simulink model "sk_R3GDL"  (Simulink 9.0)
settings: Solver=ode45  StartTime=0.0  StopTime=Tsim  MaxStep=1e-3  RelTol=1e-3  EnableMultiTasking=on
values from neighbouring files (symbols this model uses):
  A_a = [0.1 0.1 0.1]    [Estimacion_de_Parametros.m]
  A_b = [0.5 0.5 0.5]    [Estimacion_de_Parametros.m]
  Im_cc = [0 1 0.5]    [Estimacion_de_Parametros.m]
  R1 = 50    [Estimacion_de_Parametros.m]
  R2 = 30    [Estimacion_de_Parametros.m]
  R3 = 15    [Estimacion_de_Parametros.m]
  tau = 7    [Estimacion_de_Parametros.m]
  Ts = 0.001    [Estimacion_de_Parametros.m]
  W_a = [15 15 15]    [Estimacion_de_Parametros.m]
  W_b = [3 6 6]    [Estimacion_de_Parametros.m]
settings Model: Creator=mortega  LastModifiedBy=Alvaro  ExtModeTrigMode=oneshot  ExtModeArmWhenConnect=off
settings DataIOCC: SignalLoggingSaveFormat=ModelDataLogs
settings OptimizationCC: BlockReduction=off  BooleanDataType=off  ExpressionDepthLimit=2147483647  InitFltsAndDblsToZero=on
settings DebuggingCC: SaveWithParameterizedLinksMsg=none  SignalResolutionControl=TryResolveAllWithWarning  MultiTaskDSMMsg=warning  MultiTaskCondExecSysMsg=none  FcnCallInpInsideContextMsg=warning  StateNameClashWarn=warning  StrictBusMsg=None
settings HardwareCC: TargetUnknown=on
settings GRTTargetCC: TargetFcnLib=ansi_tfl_tmw.mat  CombineOutputUpdateFcns=off  GRTInterface=on

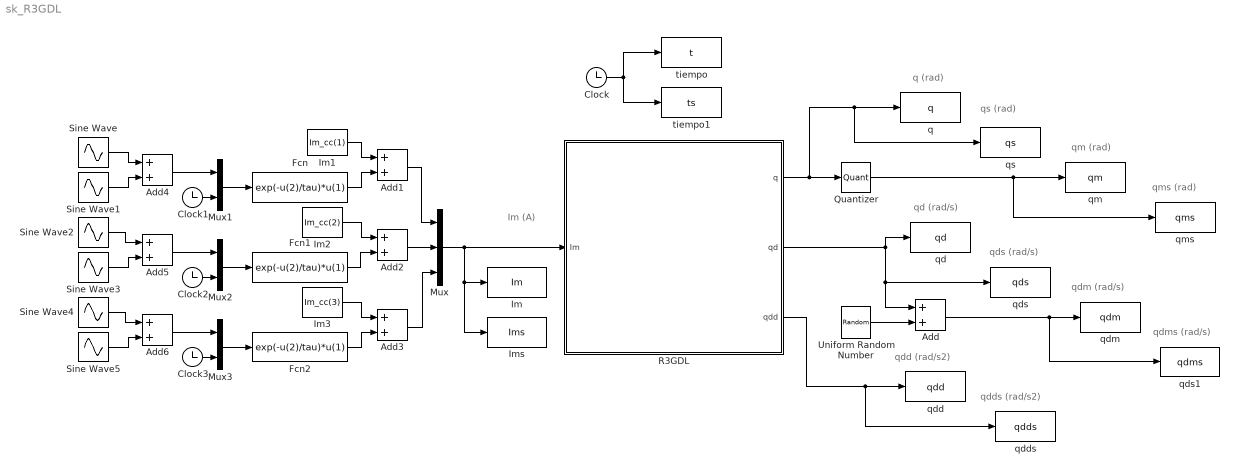
== system sk_R3GDL ==
  note: Im (A)
  note: q (rad)
  note: qd (rad/s)
  note: qdd (rad/s2)
  note: qs (rad)
  note: qds (rad/s)
  note: qdds (rad/s2)
  note: qm (rad)
  note: qms (rad)
  note: qdm (rad/s)
  note: qdms (rad/s)
  Add{,1..6} (7 alike) : Sum
  Clock{,1..3} (4 alike) : Clock
  Fcn : Fcn  Expr=exp(-u(2)/tau)*u(1)
  Fcn1 : Fcn  Expr=exp(-u(2)/tau)*u(1)
  Fcn2 : Fcn  Expr=exp(-u(2)/tau)*u(1)
  Im : ToWorkspace  VariableName=Im  SampleTime=-1
  Im1 : Constant  Value=Im_cc(1)
  Im2 : Constant  Value=Im_cc(2)
  Im3 : Constant  Value=Im_cc(3)
  Ims : ToWorkspace  VariableName=Ims  SampleTime=Ts
  Mux : Mux  Inputs=3
  Mux1 : Mux  Inputs=2
  Mux2 : Mux  Inputs=2
  Mux3 : Mux  Inputs=2
  Quantizer : Quantizer  QuantizationInterval=2*pi/512./[R1 R2 R3]
  R3GDL : Subsystem  mask(Control y Programación de Robots (4 GIERM)){NGrupo=3, q1_ini=0, q2_ini=0, q3_ini=0, Bl_q1=off, Bl_q2=off, Bl_q3=off, AccionamientoDirecto=off}
      mask prompts: NGrupo "Nº de GRUPO"; q1_ini "q1 inicial  (rad)"; q2_ini "q2 inicial (rad)"; q3_ini "q3_inicial (rad)"; Bl_q1 "Bloqueo q1"; Bl_q2 "Bloqueo q2"; Bl_q3 "Bloqueo q3"; AccionamientoDirecto "Accionamiento directo"
      mask help: Robot de 3 grados de libertad RRR
      mask Display:
      | image(imread('R3GDL_RRR.JPG'));
      | port_label('output', 1, 'q');
      | port_label('output', 2, 'qd');
      | port_label('output', 3, 'qdd');
      | port_label('input', 1, 'Im')
  Sine Wave : Sin  Amplitude=A_a(1)  Frequency=W_a(1)  SampleTime=0
  Sine Wave1 : Sin  Amplitude=A_b(1)  Frequency=W_b(1)  SampleTime=0
  Sine Wave2 : Sin  Amplitude=A_a(2)  Frequency=W_a(2)  SampleTime=0
  Sine Wave3 : Sin  Amplitude=A_b(2)  Frequency=W_b(2)  SampleTime=0
  Sine Wave4 : Sin  Amplitude=A_a(3)  Frequency=W_a(3)  SampleTime=0
  Sine Wave5 : Sin  Amplitude=A_b(3)  Frequency=W_b(3)  SampleTime=0
  Uniform Random Number : UniformRandomNumber  Minimum=-1500*2*pi/60./[R1 R2 R3]*0.02  Maximum=1500*2*pi/60./[R1 R2 R3]*0.02  SampleTime=Ts/10
  q : ToWorkspace  VariableName=q  SampleTime=-1
  qd : ToWorkspace  VariableName=qd  SampleTime=-1
  qdd : ToWorkspace  VariableName=qdd  SampleTime=-1
  qdds : ToWorkspace  VariableName=qdds  SampleTime=Ts
  qdm : ToWorkspace  VariableName=qdm  SampleTime=-1
  qds : ToWorkspace  VariableName=qds  SampleTime=Ts
  qds1 : ToWorkspace  VariableName=qdms  SampleTime=Ts
  qm : ToWorkspace  VariableName=qm  SampleTime=-1
  qms : ToWorkspace  VariableName=qms  SampleTime=Ts
  qs : ToWorkspace  VariableName=qs  SampleTime=Ts
  tiempo : ToWorkspace  VariableName=t  SampleTime=-1
  tiempo1 : ToWorkspace  VariableName=ts  SampleTime=Ts
  wires:
  Clock/1 -> tiempo1/1, tiempo/1
  Mux/1 -> Im/1, Ims/1, R3GDL/1(Im)
  R3GDL/1(q) -> qs/1, q/1, Quantizer/1
  R3GDL/2(qd) -> qd/1, Add/1, qds/1
  R3GDL/3(qdd) -> qdds/1, qdd/1
  Quantizer/1 -> qms/1, qm/1
  Uniform Random Number/1 -> Add/2
  Add/1 -> qds1/1, qdm/1
  Im1/1 -> Add1/1
  Fcn/1 -> Add1/2
  Add1/1 -> Mux/1
  Fcn1/1 -> Add2/2
  Im2/1 -> Add2/1
  Add2/1 -> Mux/2
  Im3/1 -> Add3/1
  Fcn2/1 -> Add3/2
  Add3/1 -> Mux/3
  Mux1/1 -> Fcn/1
  Mux2/1 -> Fcn1/1
  Mux3/1 -> Fcn2/1
  Clock1/1 -> Mux1/2
  Clock2/1 -> Mux2/2
  Clock3/1 -> Mux3/2
  Add4/1 -> Mux1/1
  Add5/1 -> Mux2/1
  Add6/1 -> Mux3/1
  Sine Wave/1 -> Add4/1
  Sine Wave1/1 -> Add4/2
  Sine Wave2/1 -> Add5/1
  Sine Wave3/1 -> Add5/2
  Sine Wave4/1 -> Add6/1
  Sine Wave5/1 -> Add6/2

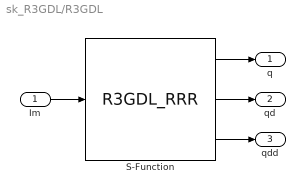
== system sk_R3GDL/R3GDL ==
  Im : Inport
  S-Function : S-Function  FunctionName=R3GDL_RRR  Parameters=[q1_ini; q2_ini; q3_ini]; [Bl_q1; Bl_q2; Bl_q3]; AccionamientoDirecto; NGrupo  SFunctionDeploymentMode=off  EnableBusSupport=off
  q : Outport
  qd : Outport  Port=2
  qdd : Outport  Port=3
  wires:
  Im/1 -> S-Function/1
  S-Function/1 -> q/1
  S-Function/2 -> qd/1
  S-Function/3 -> qdd/1
